simulink model "hevmodel"  (R2016b)
settings: Solver=VariableStepAuto  StartTime=0.0  StopTime=100.0  RelTol=1e-3
undefined symbols (not defined in the file): c_b_e1, c_b_E1, c_b_E2, c_b_e3, c_b_E3, c_b_E4, c_b_L1, c_b_L2, c_b_L3, c_b_L4, F, G, h, H_l, I_b_max, Mz, N, Q1, Q2, Q_b_0, rho_f, Ts, ubounds, w_eg_upper, w_em_upper, w_ice_upper
settings Model: Creator=Niklas  LastModifiedBy=Niklas
settings DataIOCC: SaveTime=off

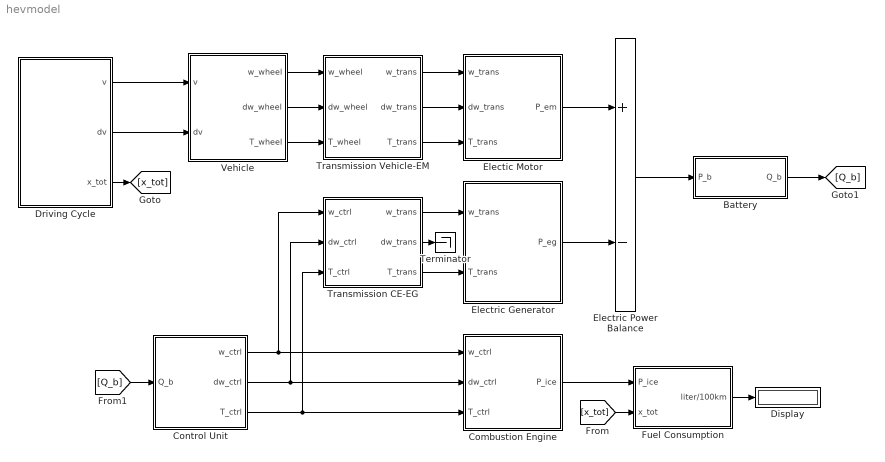
== system hevmodel ==
  Battery : Subsystem  mask{I_0=80, Q_b_IC_rel=50, t_ch=20}
      mask prompts: I_0 "Energy capacity of battery [Ah]"; Q_b_IC_rel "Initial charge of battery [%]"; t_ch "Current limit: minimum time to charge/discharge the battery [min]"
      mask init:
      | init_battery;
  Combustion Engine : Subsystem  mask{theta_ice=1, H_l=1, w_ice_idle=1, T_ice_idle=1, P_ice_idle=1, ENABLE_FUEL_CUTOFF=0, T_ice_cutoff=0, P_ice_cutoff=0}
      mask prompts: theta_ice "Engine inertia [kg*m^2]"; H_l "Fuel's lower heating value []"; w_ice_idle "Engine speed at idle [rad/s]"; T_ice_idle "Engine torque at idle [Nm]"; P_ice_idle "Engine power at idle [W]"; ENABLE_FUEL_CUTOFF "Enable fuel cutoff"; T_ice_cutoff "Engine torque at fuel cutoff [Nm]"; P_ice_cutoff "Engine power at fuel cutoff [W]"
  Control Unit : Subsystem
  Display : Display
  Driving Cycle : Subsystem  mask{Ts=0.1}
      mask prompts: Ts "Step size [s]"
      mask init:
      | init_drive_cycle
  Electic Motor : Subsystem  mask{theta_em=1}
      mask prompts: theta_em "Motor Ineratia [kg*m^2]"
      mask init:
      | init_EM
  Electric Generator : Subsystem
  Electric Power Balance : Sum  Inputs=+-
  Fuel Consumption : Subsystem
      mask init:
      | init_tank;
  Terminator : Terminator
  Transmission CE-EG : Subsystem  mask{gear_ratio=1, eta_gb=1, P_gb0=0, w_wheel_min=1}
      mask prompts: gear_ratio "Gear Ratio"; eta_gb "Efficiency"; P_gb0 "Idling losses (friction) [W]"; w_wheel_min "Minimum wheel speed beyond which losses are generated [rad/s]"
      mask init:
      | init_transmission;
  Transmission Vehicle-EM : Subsystem  mask{gear_ratio=0.707, eta_gb=0.975, P_gb0=0, w_wheel_min=1}
      mask prompts: gear_ratio "Gear Ratio"; eta_gb "Efficiency"; P_gb0 "Idling losses (friction) [W]"; w_wheel_min "Minimum wheel speed beyond which losses are generated [rad/s]"
      mask init:
      | init_transmission;
  Vehicle : Subsystem  mask{r_wheel=0.82, R0=554.9, R1=20.3, R2=3.56}
      mask prompts: r_wheel "Wheel Radius [m]"; R0 "Running Resistance R0 [N]"; R1 "Running Resistance R1 [N/(m/s)]"; R2 "Running Resistance R2 [N/(m/s)^2]"
      mask init:
      | init_vehicle
  wires:
  Transmission Vehicle-EM/1(w_trans) -> Electic Motor/1(w_trans)
  Transmission Vehicle-EM/2(dw_trans) -> Electic Motor/2(dw_trans)
  Transmission Vehicle-EM/3(T_trans) -> Electic Motor/3(T_trans)
  Vehicle/1(w_wheel) -> Transmission Vehicle-EM/1(w_wheel)
  Vehicle/2(dw_wheel) -> Transmission Vehicle-EM/2(dw_wheel)
  Vehicle/3(T_wheel) -> Transmission Vehicle-EM/3(T_wheel)
  Control Unit/1(w_ctrl) -> Transmission CE-EG/1(w_ctrl), Combustion Engine/1(w_ctrl)
  Control Unit/3(T_ctrl) -> Transmission CE-EG/3(T_ctrl), Combustion Engine/3(T_ctrl)
  Combustion Engine/1(P_ice) -> Fuel Consumption/1(P_ice)
  Fuel Consumption/1(liter/100km) -> Display/1
  Control Unit/2(dw_ctrl) -> Transmission CE-EG/2(dw_ctrl), Combustion Engine/2(dw_ctrl)
  Driving Cycle/1(v) -> Vehicle/1(v)
  Driving Cycle/2(dv) -> Vehicle/2(dv)
  Electric Power Balance/1 -> Battery/1(P_b)
  Electic Motor/1(P_em) -> Electric Power Balance/1
  Electric Generator/1(P_eg) -> Electric Power Balance/2
  Transmission CE-EG/1(w_trans) -> Electric Generator/1(w_trans)
  Transmission CE-EG/3(T_trans) -> Electric Generator/2(T_trans)
  Transmission CE-EG/2(dw_trans) -> Terminator/1
  Driving Cycle/3(x_tot) -> [x_tot]
  [x_tot] -> Fuel Consumption/2(x_tot)
  Battery/1(Q_b) -> [Q_b]
  [Q_b] -> Control Unit/1(Q_b)

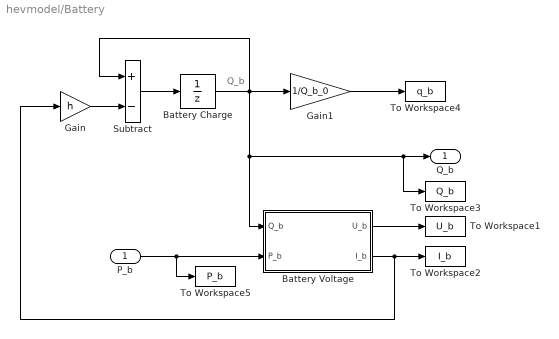
== system hevmodel/Battery ==
  note: Q_b
  P_b : Inport
  Battery Charge : UnitDelay  SampleTime=-1
  Battery Voltage : Subsystem
  Gain : Gain  Gain=h
  Gain1 : Gain  Gain=1/Q_b_0
  Subtract : Sum  Inputs=+-
  To Workspace1 : ToWorkspace  VariableName=U_b  SaveFormat=Timeseries  SampleTime=-1
  To Workspace2 : ToWorkspace  VariableName=I_b  SaveFormat=Timeseries  SampleTime=-1
  To Workspace3 : ToWorkspace  VariableName=Q_b  SaveFormat=Timeseries  SampleTime=-1
  To Workspace4 : ToWorkspace  VariableName=q_b  SaveFormat=Timeseries  SampleTime=-1
  To Workspace5 : ToWorkspace  VariableName=P_b  SaveFormat=Timeseries  SampleTime=-1
  Q_b : Outport
  wires:
  P_b/1 -> To Workspace5/1, Battery Voltage/2(P_b)
  Battery Charge/1 -> Subtract/1, Gain1/1, Battery Voltage/1(Q_b), To Workspace3/1, Q_b/1
  Subtract/1 -> Battery Charge/1
  Gain/1 -> Subtract/2
  Battery Voltage/2(I_b) -> To Workspace2/1, Gain/1
  Battery Voltage/1(U_b) -> To Workspace1/1
  Gain1/1 -> To Workspace4/1

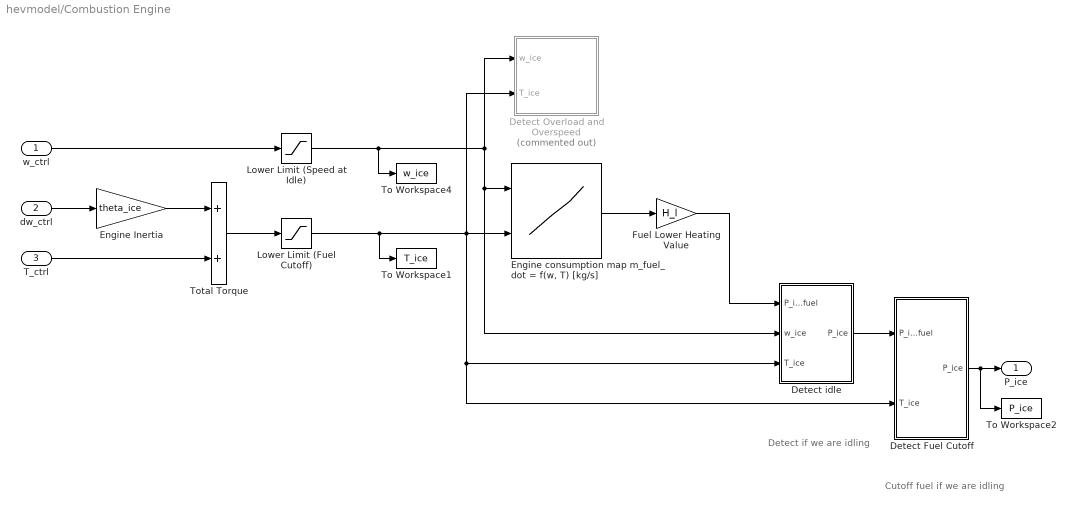
== system hevmodel/Combustion Engine ==
  note: Detect if we are idling
  note: Cutoff fuel if we are idling
  w_ctrl : Inport
  dw_ctrl : Inport  Port=2
  T_ctrl : Inport  Port=3
  Detect Fuel Cutoff : Subsystem
  Detect Overload and Overspeed : Subsystem  Commented=on
  Detect idle : Subsystem
  Engine Inertia : Gain  Gain=theta_ice
  "Engine consumption map m_fuel_dot = f(w, T) [kg/s]" : Lookup_n-D  BreakpointsForDimension1=[1:3]  BreakpointsForDimension2=[1:3]  InternalRulePriority=Speed  RndMeth=Simplest  InputSameDT=on
  Fuel Lower Heating Value : Gain  Gain=H_l
  Lower Limit (Fuel Cutoff) : Saturate  UpperLimit=inf  LowerLimit=T_ice_cutoff
  Lower Limit (Speed at Idle) : Saturate  UpperLimit=inf  LowerLimit=w_ice_idle
  To Workspace1 : ToWorkspace  VariableName=T_ice  SaveFormat=Timeseries  SampleTime=-1
  To Workspace2 : ToWorkspace  VariableName=P_ice  SaveFormat=Timeseries  SampleTime=-1
  To Workspace4 : ToWorkspace  VariableName=w_ice  SaveFormat=Timeseries  SampleTime=-1
  Total Torque : Sum
  P_ice : Outport
  wires:
  Detect Fuel Cutoff/1(P_ice) -> To Workspace2/1, P_ice/1
  dw_ctrl/1 -> Engine Inertia/1
  Engine Inertia/1 -> Total Torque/1
  T_ctrl/1 -> Total Torque/2
  Total Torque/1 -> Lower Limit (Fuel Cutoff)/1
  w_ctrl/1 -> Lower Limit (Speed at Idle)/1
  Lower Limit (Fuel Cutoff)/1 -> To Workspace1/1, Detect Overload and Overspeed/2(T_ice), Detect idle/3(T_ice), Detect Fuel Cutoff/2(T_ice), "Engine consumption map m_fuel_dot = f(w, T) [kg/s]"/2
  "Engine consumption map m_fuel_dot = f(w, T) [kg/s]"/1 -> Fuel Lower Heating Value/1
  Fuel Lower Heating Value/1 -> Detect idle/1(P_ice_fuel)
  Detect idle/1(P_ice) -> Detect Fuel Cutoff/1(P_ice_fuel)
  Lower Limit (Speed at Idle)/1 -> To Workspace4/1, Detect idle/2(w_ice), "Engine consumption map m_fuel_dot = f(w, T) [kg/s]"/1, Detect Overload and Overspeed/1(w_ice)

== system hevmodel/Control Unit ==
  Q_b : Inport
  Constant : Constant  Value=0
  MPC Controller : Subsystem  Commented=on  mask{F=F, G=G, M=Mz, N=N, Q1=Q1, Q2=Q2, ubounds=ubounds, Ts=Ts, ufname='solvempcproblem'}
      mask prompts: ubounds "Input bounds [u1min u1max;u2min u2max;...]"; ufname "Output function (Ex: 'myfun1')"
      mask Display:
      | port_label('input',1,'x')
      | port_label('output',1,'u')
  Terminator : Terminator
  w_ctrl : Outport
  dw_ctrl : Outport  Port=2
  T_ctrl : Outport  Port=3
  wires:
  Constant/1 -> T_ctrl/1, w_ctrl/1, dw_ctrl/1
  Q_b/1 -> Terminator/1

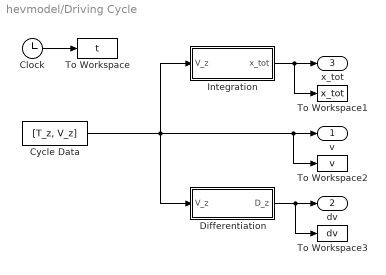
== system hevmodel/Driving Cycle ==
  Clock : Clock
  Cycle Data : FromWorkspace  VariableName=[T_z, V_z]  SampleTime=h
  Differentiation : Subsystem
  Integration : Subsystem
  To Workspace : ToWorkspace  VariableName=t  SampleTime=h
  To Workspace1 : ToWorkspace  VariableName=x_tot  SampleTime=-1
  To Workspace2 : ToWorkspace  VariableName=v  SampleTime=-1
  To Workspace3 : ToWorkspace  VariableName=dv  SampleTime=-1
  v : Outport
  dv : Outport  Port=2
  x_tot : Outport  Port=3
  wires:
  Clock/1 -> To Workspace/1
  Cycle Data/1 -> Differentiation/1(V_z), Integration/1(V_z), To Workspace2/1, v/1
  Integration/1(x_tot) -> To Workspace1/1, x_tot/1
  Differentiation/1(D_z) -> To Workspace3/1, dv/1

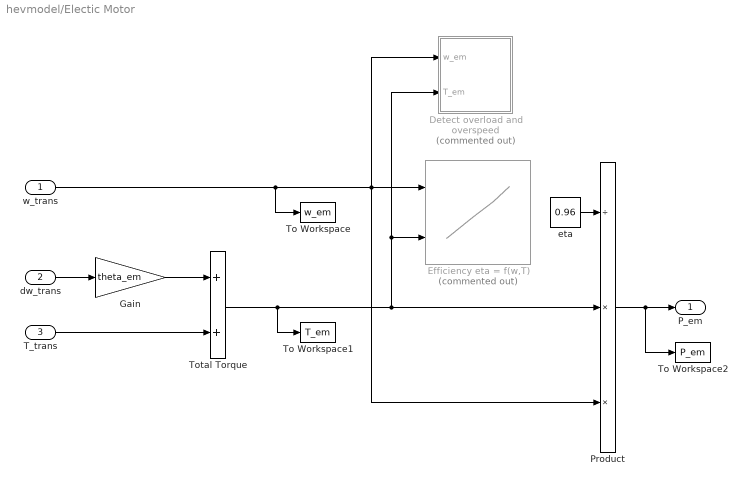
== system hevmodel/Electic Motor ==
  w_trans : Inport
  dw_trans : Inport  Port=2
  T_trans : Inport  Port=3
  Detect overload and overspeed : Subsystem  Commented=on
  Efficiency eta = f(w,T) : Lookup_n-D  Commented=on  BreakpointsForDimension1=[1:3]  BreakpointsForDimension2=[1:3]  InternalRulePriority=Speed  RndMeth=Simplest  InputSameDT=on
  Gain : Gain  Gain=theta_em
  Product : Product  Inputs=/**
  To Workspace : ToWorkspace  VariableName=w_em  SaveFormat=Timeseries  SampleTime=-1
  To Workspace1 : ToWorkspace  VariableName=T_em  SaveFormat=Timeseries  SampleTime=-1
  To Workspace2 : ToWorkspace  VariableName=P_em  SaveFormat=Timeseries  SampleTime=-1
  Total Torque : Sum
  eta : Constant  Value=0.96
  P_em : Outport
  wires:
  Product/1 -> To Workspace2/1, P_em/1
  dw_trans/1 -> Gain/1
  Gain/1 -> Total Torque/1
  T_trans/1 -> Total Torque/2
  Total Torque/1 -> To Workspace1/1, Efficiency eta = f(w,T)/2, Detect overload and overspeed/2(T_em), Product/2
  w_trans/1 -> To Workspace/1, Product/3, Detect overload and overspeed/1(w_em), Efficiency eta = f(w,T)/1
  eta/1 -> Product/1

== system hevmodel/Electric Generator ==
  w_trans : Inport
  T_trans : Inport  Port=2
  Detect overload and overspeed : Subsystem  Commented=on
  Efficiency eta = f(w,T) : Lookup_n-D  Commented=on  BreakpointsForDimension1=[1:3]  BreakpointsForDimension2=[1:3]  InternalRulePriority=Speed  RndMeth=Simplest  InputSameDT=on
  Product : Product  Inputs=3
  To Workspace1 : ToWorkspace  VariableName=w_eg  SaveFormat=Timeseries  SampleTime=-1
  To Workspace2 : ToWorkspace  VariableName=T_eg  SaveFormat=Timeseries  SampleTime=-1
  To Workspace3 : ToWorkspace  VariableName=P_eg  SaveFormat=Timeseries  SampleTime=-1
  eta : Constant  Value=0.96
  P_eg : Outport
  wires:
  Product/1 -> To Workspace3/1, P_eg/1
  T_trans/1 -> To Workspace2/1, Efficiency eta = f(w,T)/2, Detect overload and overspeed/2(T_eg), Product/2
  w_trans/1 -> To Workspace1/1, Product/3, Detect overload and overspeed/1(w_eg), Efficiency eta = f(w,T)/1
  eta/1 -> Product/1

== system hevmodel/Fuel Consumption ==
  P_ice : Inport
  x_tot : Inport  Port=2
  Divide : Product  Inputs=*/
  Gain : Gain  Gain=1/rho_f
  Gain1 : Gain  Gain=1e5
  Integration : Subsystem
  Saturation : Saturate  UpperLimit=inf  LowerLimit=1
  liter/100km : Outport
  wires:
  P_ice/1 -> Integration/1(P_ice)
  Gain1/1 -> liter/100km/1
  Integration/1(m_fuel) -> Gain/1
  Gain/1 -> Divide/1
  Divide/1 -> Gain1/1
  x_tot/1 -> Saturation/1
  Saturation/1 -> Divide/2

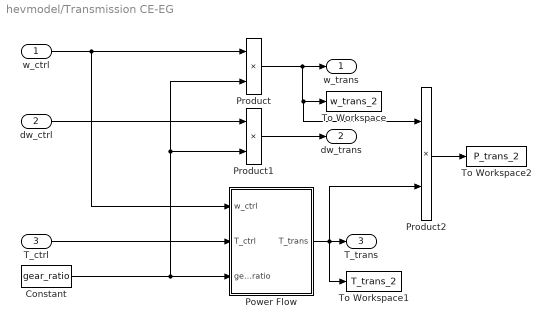
== system hevmodel/Transmission CE-EG ==
  w_ctrl : Inport
  dw_ctrl : Inport  Port=2
  T_ctrl : Inport  Port=3
  Constant : Constant  Value=gear_ratio
  Power Flow : Subsystem
  Product : Product
  Product1 : Product
  Product2 : Product
  To Workspace : ToWorkspace  VariableName=w_trans_2  SaveFormat=Timeseries  SampleTime=-1
  To Workspace1 : ToWorkspace  VariableName=T_trans_2  SaveFormat=Timeseries  SampleTime=-1
  To Workspace2 : ToWorkspace  VariableName=P_trans_2  SaveFormat=Timeseries  SampleTime=-1
  w_trans : Outport
  dw_trans : Outport  Port=2
  T_trans : Outport  Port=3
  wires:
  w_ctrl/1 -> Product/1, Power Flow/1(w_ctrl)
  dw_ctrl/1 -> Product1/1
  Product/1 -> Product2/1, To Workspace/1, w_trans/1
  Power Flow/1(T_trans) -> To Workspace1/1, Product2/2, T_trans/1
  Product1/1 -> dw_trans/1
  T_ctrl/1 -> Power Flow/2(T_ctrl)
  Constant/1 -> Product/2, Product1/2, Power Flow/3(gear_ratio)
  Product2/1 -> To Workspace2/1

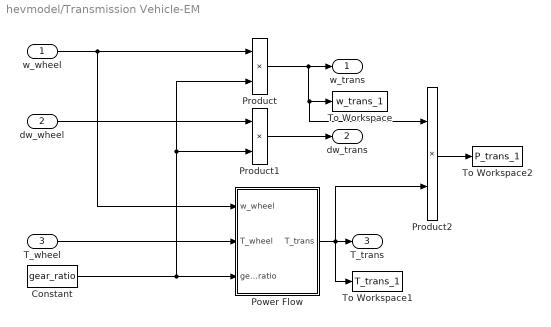
== system hevmodel/Transmission Vehicle-EM ==
  w_wheel : Inport
  dw_wheel : Inport  Port=2
  T_wheel : Inport  Port=3
  Constant : Constant  Value=gear_ratio
  Power Flow : Subsystem
  Product : Product
  Product1 : Product
  Product2 : Product
  To Workspace : ToWorkspace  VariableName=w_trans_1  SaveFormat=Timeseries  SampleTime=-1
  To Workspace1 : ToWorkspace  VariableName=T_trans_1  SaveFormat=Timeseries  SampleTime=-1
  To Workspace2 : ToWorkspace  VariableName=P_trans_1  SaveFormat=Timeseries  SampleTime=-1
  w_trans : Outport
  dw_trans : Outport  Port=2
  T_trans : Outport  Port=3
  wires:
  w_wheel/1 -> Product/1, Power Flow/1(w_wheel)
  dw_wheel/1 -> Product1/1
  Product/1 -> Product2/1, To Workspace/1, w_trans/1
  Power Flow/1(T_trans) -> To Workspace1/1, Product2/2, T_trans/1
  Product1/1 -> dw_trans/1
  T_wheel/1 -> Power Flow/2(T_wheel)
  Constant/1 -> Product/2, Product1/2, Power Flow/3(gear_ratio)
  Product2/1 -> To Workspace2/1

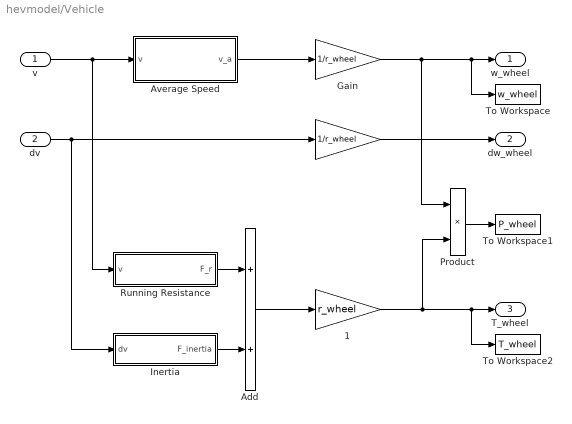
== system hevmodel/Vehicle ==
  v : Inport
  dv : Inport  Port=2
  " " : Gain  Gain=1/r_wheel
  " 1" : Gain  Gain=r_wheel
  Add : Sum
  Average Speed : Subsystem
  Gain : Gain  Gain=1/r_wheel
  Inertia : Subsystem
  Product : Product
  Running Resistance : Subsystem
  To Workspace : ToWorkspace  VariableName=w_wheel  SaveFormat=Timeseries  SampleTime=-1
  To Workspace1 : ToWorkspace  VariableName=P_wheel  SaveFormat=Timeseries  SampleTime=-1
  To Workspace2 : ToWorkspace  VariableName=T_wheel  SaveFormat=Timeseries  SampleTime=-1
  w_wheel : Outport
  dw_wheel : Outport  Port=2
  T_wheel : Outport  Port=3
  wires:
  v/1 -> Running Resistance/1(v), Average Speed/1(v)
  Gain/1 -> To Workspace/1, w_wheel/1, Product/1
  " "/1 -> dw_wheel/1
  dv/1 -> Inertia/1(dv), " "/1
  " 1"/1 -> To Workspace2/1, T_wheel/1, Product/2
  Product/1 -> To Workspace1/1
  Average Speed/1(v_a) -> Gain/1
  Add/1 -> " 1"/1
  Inertia/1(F_inertia) -> Add/2
  Running Resistance/1(F_r) -> Add/1

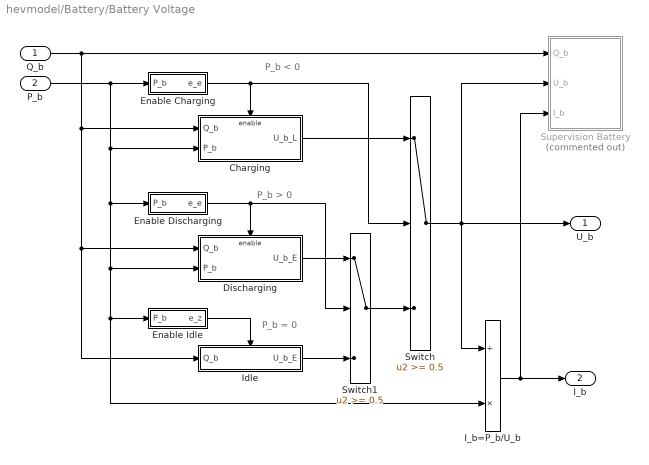
== system hevmodel/Battery/Battery Voltage ==
  note: P_b < 0
  note: P_b = 0
  note: P_b > 0
  Q_b : Inport
  P_b : Inport  Port=2
  Charging : Subsystem
  Discharging : Subsystem
  Enable Charging : Subsystem
  Enable Discharging : Subsystem
  Enable Idle : Subsystem
  I_b=P_b/U_b : Product  Inputs=/*
  Idle : Subsystem
  Supervision Battery : Subsystem  Commented=on
  Switch : Switch  Threshold=0.5
  Switch1 : Switch  Threshold=0.5
  U_b : Outport
  I_b : Outport  Port=2
  wires:
  Q_b/1 -> Charging/1(Q_b), Idle/1(Q_b), Discharging/1(Q_b), Supervision Battery/1(Q_b)
  Enable Charging/1(e_e) -> Switch/2, Charging/Enable
  I_b=P_b/U_b/1 -> I_b/1, Supervision Battery/3(I_b)
  P_b/1 -> I_b=P_b/U_b/2, Enable Idle/1(P_b), Discharging/2(P_b), Enable Discharging/1(P_b), Charging/2(P_b), Enable Charging/1(P_b)
  Enable Idle/1(e_z) -> Idle/Enable
  Enable Discharging/1(e_e) -> Switch1/2, Discharging/Enable
  Discharging/1(U_b_E) -> Switch1/1
  Switch1/1 -> Switch/3
  Idle/1(U_b_E) -> Switch1/3
  Switch/1 -> I_b=P_b/U_b/1, Supervision Battery/2(U_b), U_b/1
  Charging/1(U_b_L) -> Switch/1

== system hevmodel/Combustion Engine/Detect Fuel Cutoff ==
  P_ice_fuel : Inport
  T_ice : Inport  Port=2
  Constant : Constant  Value=P_ice_cutoff
  Constant1 : Constant  Value=ENABLE_FUEL_CUTOFF
  Switch1 : Switch  Threshold=T_ice_cutoff + 0.01
  Switch2 : Switch  Threshold=0.5
  P_ice : Outport
  wires:
  Switch2/1 -> P_ice/1
  T_ice/1 -> Switch1/2
  P_ice_fuel/1 -> Switch2/3, Switch1/1
  Constant/1 -> Switch1/3
  Constant1/1 -> Switch2/2
  Switch1/1 -> Switch2/1

== system hevmodel/Combustion Engine/Detect Overload and Overspeed ==
  w_ice : Inport
  T_ice : Inport  Port=2
  Abs : Abs
  Constant : Constant  Value=w_ice_upper
  Maximum Torque : Lookup_n-D  NumberOfTableDimensions=1  BreakpointsForDimension1=[-5:5]  Table=tanh([-5:5])  InternalRulePriority=Speed  RndMeth=Simplest  InputSameDT=on
  Saturation : Saturate  UpperLimit=0  LowerLimit=-inf
  Saturation1 : Saturate  UpperLimit=0  LowerLimit=-inf
  Stop Simulation : Stop
  Stop Simulation1 : Stop
  Subtract1 : Sum  Inputs=+-
  Subtract2 : Sum  Inputs=+-
  wires:
  Maximum Torque/1 -> Subtract1/1
  Subtract1/1 -> Saturation/1
  Saturation/1 -> Stop Simulation/1
  Abs/1 -> Subtract1/2
  w_ice/1 -> Subtract2/2, Maximum Torque/1
  T_ice/1 -> Abs/1
  Constant/1 -> Subtract2/1
  Saturation1/1 -> Stop Simulation1/1
  Subtract2/1 -> Saturation1/1

== system hevmodel/Combustion Engine/Detect idle ==
  P_ice_fuel : Inport
  w_ice : Inport  Port=2
  T_ice : Inport  Port=3
  Constant : Constant  Value=P_ice_idle
  Idle detection : Fcn  Expr=(u(1) <= w_ice_idle) * (u(2) <= T_ice_idle)
  Mux : Mux  Inputs=2
  Switch : Switch  Criteria=u2 > Threshold
  P_ice : Outport
  wires:
  w_ice/1 -> Mux/1
  T_ice/1 -> Mux/2
  Switch/1 -> P_ice/1
  P_ice_fuel/1 -> Switch/3
  Constant/1 -> Switch/1
  Idle detection/1 -> Switch/2
  Mux/1 -> Idle detection/1

== system hevmodel/Control Unit/MPC Controller ==
  In1 : Inport
  Clock : Clock
  MPC Controller1 : M-S-Function  FunctionName=mympccontroller  Parameters=F,G,M,N,Q1,Q2,ubounds,Ts,ufname  mask{F=F, G=G, M=M, N=N, Q1=Q1, Q2=Q2, ubounds=ubounds, Ts=Ts, ufname=ufname}
      mask prompts: ubounds "ubounds [u1min u1max;u2min u2max;...]"; ufname "Output function (Ex: 'myfun1')"
      mask Display:
      | port_label('input',1,'x')
      | port_label('input',2,'t')
      | port_label('output',1,'u')
  Out1 : Outport
  wires:
  Clock/1 -> MPC Controller1/2
  In1/1 -> MPC Controller1/1
  MPC Controller1/1 -> Out1/1

== system hevmodel/Driving Cycle/Differentiation ==
  V_z : Inport
  Add : Sum  Inputs=+-
  Unit Delay : UnitDelay  SampleTime=-1
  D_z : Outport
  wires:
  Unit Delay/1 -> Add/2
  V_z/1 -> Unit Delay/1, Add/1
  Add/1 -> D_z/1

== system hevmodel/Driving Cycle/Integration ==
  V_z : Inport
  Add : Sum
  Add1 : Sum
  Gain : Gain  Gain=0.5*h
  Unit Delay : UnitDelay  SampleTime=-1
  Unit Delay1 : UnitDelay  SampleTime=-1
  x_tot : Outport
  wires:
  Unit Delay/1 -> Add/2
  V_z/1 -> Add/1, Unit Delay/1
  Add/1 -> Gain/1
  Gain/1 -> Add1/2
  Add1/1 -> Unit Delay1/1
  Unit Delay1/1 -> x_tot/1, Add1/1

== system hevmodel/Electic Motor/Detect overload and overspeed ==
  w_em : Inport
  T_em : Inport  Port=2
  Abs : Abs
  Add : Sum  Inputs=+-
  Add1 : Sum  Inputs=+-
  Constant : Constant  Value=w_em_upper
  Maximum Torque : Lookup_n-D  NumberOfTableDimensions=1  BreakpointsForDimension1=[-5:5]  Table=tanh([-5:5])  InternalRulePriority=Speed  RndMeth=Simplest  InputSameDT=on
  Saturation : Saturate  UpperLimit=0  LowerLimit=-inf
  Saturation1 : Saturate  UpperLimit=0  LowerLimit=-inf
  Stop Simulation : Stop
  Stop Simulation1 : Stop
  wires:
  w_em/1 -> Add1/2, Maximum Torque/1
  T_em/1 -> Abs/1
  Maximum Torque/1 -> Add/1
  Abs/1 -> Add/2
  Add/1 -> Saturation/1
  Saturation/1 -> Stop Simulation1/1
  Constant/1 -> Add1/1
  Add1/1 -> Saturation1/1
  Saturation1/1 -> Stop Simulation/1

== system hevmodel/Electric Generator/Detect overload and overspeed ==
  w_eg : Inport
  T_eg : Inport  Port=2
  Abs : Abs
  Add : Sum  Inputs=+-
  Add1 : Sum  Inputs=+-
  Constant : Constant  Value=w_eg_upper
  Maximum Torque : Lookup_n-D  NumberOfTableDimensions=1  BreakpointsForDimension1=[-5:5]  Table=tanh([-5:5])  InternalRulePriority=Speed  RndMeth=Simplest  InputSameDT=on
  Saturation : Saturate  UpperLimit=0  LowerLimit=-inf
  Saturation1 : Saturate  UpperLimit=0  LowerLimit=-inf
  Stop Simulation : Stop
  Stop Simulation1 : Stop
  wires:
  w_eg/1 -> Add1/2, Maximum Torque/1
  T_eg/1 -> Abs/1
  Maximum Torque/1 -> Add/1
  Abs/1 -> Add/2
  Add/1 -> Saturation/1
  Saturation/1 -> Stop Simulation1/1
  Constant/1 -> Add1/1
  Add1/1 -> Saturation1/1
  Saturation1/1 -> Stop Simulation/1

== system hevmodel/Fuel Consumption/Integration ==
  P_ice : Inport
  Add1 : Sum
  Add2 : Sum
  Constant : Constant  Value=1/H_l
  Fuel Consumption : UnitDelay  SampleTime=-1
  Gain : Gain  Gain=0.5*h
  Product : Product
  To Workspace1 : ToWorkspace  VariableName=m_dot_fuel  SaveFormat=Timeseries  SampleTime=-1
  To Workspace2 : ToWorkspace  VariableName=m_fuel  SaveFormat=Timeseries  SampleTime=-1
  Unit Delay : UnitDelay  SampleTime=-1
  m_fuel : Outport
  wires:
  Fuel Consumption/1 -> To Workspace2/1, m_fuel/1, Add1/1
  Add1/1 -> Fuel Consumption/1
  P_ice/1 -> Add2/1, Unit Delay/1
  Unit Delay/1 -> Add2/2
  Constant/1 -> Product/1
  Add2/1 -> Gain/1
  Gain/1 -> Product/2
  Product/1 -> To Workspace1/1, Add1/2

== system hevmodel/Transmission CE-EG/Power Flow ==
  w_ctrl : Inport
  T_ctrl : Inport  Port=2
  gear_ratio : Inport  Port=3
  Subsystem : Subsystem
  Subsystem1 : Subsystem
  Switch : Switch
  T_trans : Outport
  wires:
  T_ctrl/1 -> Subsystem1/2(T_ctrl), Subsystem/2(T_ctrl), Switch/2
  Switch/1 -> T_trans/1
  Subsystem1/1(T_trans-) -> Switch/3
  Subsystem/1(T_trans+) -> Switch/1
  gear_ratio/1 -> Subsystem1/3(gear_ratio), Subsystem/3(gear_ratio)
  w_ctrl/1 -> Subsystem1/1(w_ctrl), Subsystem/1(w_ctrl)

== system hevmodel/Transmission Vehicle-EM/Power Flow ==
  w_wheel : Inport
  T_wheel : Inport  Port=2
  gear_ratio : Inport  Port=3
  "Energy Engine -> Wheel" : Subsystem
  "Energy Wheel -> Engine" : Subsystem
  Switch : Switch
  T_trans : Outport
  wires:
  T_wheel/1 -> "Energy Wheel -> Engine"/2(T_wheel), "Energy Engine -> Wheel"/2(T_wheel), Switch/2
  Switch/1 -> T_trans/1
  "Energy Wheel -> Engine"/1(T_trans-) -> Switch/3
  "Energy Engine -> Wheel"/1(T_trans+) -> Switch/1
  gear_ratio/1 -> "Energy Wheel -> Engine"/3(gear_ratio), "Energy Engine -> Wheel"/3(gear_ratio)
  w_wheel/1 -> "Energy Wheel -> Engine"/1(w_wheel), "Energy Engine -> Wheel"/1(w_wheel)

== system hevmodel/Vehicle/Average Speed ==
  v : Inport
  Add : Sum
  Gain : Gain  Gain=0.5
  Unit Delay : UnitDelay  SampleTime=-1
  v_a : Outport
  wires:
  v/1 -> Unit Delay/1, Add/1
  Unit Delay/1 -> Add/2
  Add/1 -> Gain/1
  Gain/1 -> v_a/1

== system hevmodel/Vehicle/Inertia ==
  dv : Inport
  Inertia : Fcn  Expr=39600*(1.08)*u/h
  F_inertia : Outport
  wires:
  dv/1 -> Inertia/1
  Inertia/1 -> F_inertia/1

== system hevmodel/Vehicle/Running Resistance ==
  v : Inport
  Running Resistance : Fcn  Expr=R2*u^2+R1*u+R0
  Standstill : Constant  Value=0
  Switch : Switch  Criteria=u2 > Threshold
  F_r : Outport
  wires:
  Running Resistance/1 -> Switch/1
  v/1 -> Switch/2, Running Resistance/1
  Switch/1 -> F_r/1
  Standstill/1 -> Switch/3

== system hevmodel/Battery/Battery Voltage/Charging ==
  note: P_b/I_0
  note: 1- q
  Q_b : Inport
  P_b : Inport  Port=2
  Enable : EnablePort
  Constant : Constant  Value=Q_b_0
  Fcn1 : Fcn  Expr=(c_b_L3*u[1]+c_b_L1+sqrt((c_b_L3*u[1]+c_b_L1)^2+4*(c_b_L4*u[1]+c_b_L2)*(-u[2])))/2
  Gain : Gain  Gain=1/Q_b_0
  Gain1 : Gain  Gain=1/I_0
  Mux : Mux  Inputs=2
  Subtract : Sum  Inputs=-+
  U_b_L : Outport
  wires:
  P_b/1 -> Gain1/1
  Gain1/1 -> Mux/2
  Gain/1 -> Mux/1
  Subtract/1 -> Gain/1
  Constant/1 -> Subtract/2
  Q_b/1 -> Subtract/1
  Fcn1/1 -> U_b_L/1
  Mux/1 -> Fcn1/1

== system hevmodel/Battery/Battery Voltage/Discharging ==
  note: P/I_0
  note: 1-q
  Q_b : Inport
  P_b : Inport  Port=2
  Enable : EnablePort
  Constant : Constant  Value=Q_b_0
  Fcn : Fcn  Expr=(c_b_E3*u[1]+c_b_E1+sqrt((c_b_E3*u[1]+c_b_E1)^2+4*(c_b_E4*u[1]+c_b_E2)*(-u[2])))/2
  Gain : Gain  Gain=1/Q_b_0
  Gain1 : Gain  Gain=1/I_0
  Mux : Mux  Inputs=2
  Subtract : Sum  Inputs=-+
  U_b_E : Outport
  wires:
  Gain1/1 -> Mux/2
  Gain/1 -> Mux/1
  Subtract/1 -> Gain/1
  Constant/1 -> Subtract/2
  Fcn/1 -> U_b_E/1
  Mux/1 -> Fcn/1
  Q_b/1 -> Subtract/1
  P_b/1 -> Gain1/1

== system hevmodel/Battery/Battery Voltage/Enable Charging ==
  P_b : Inport
  Gain : Gain  Gain=-1
  Saturation : Saturate  UpperLimit=0  LowerLimit=-inf
  Sign : Signum
  e_e : Outport
  wires:
  Sign/1 -> e_e/1
  P_b/1 -> Saturation/1
  Saturation/1 -> Gain/1
  Gain/1 -> Sign/1

== system hevmodel/Battery/Battery Voltage/Enable Discharging ==
  P_b : Inport
  Saturation : Saturate  UpperLimit=inf  LowerLimit=0
  Sign : Signum
  e_e : Outport
  wires:
  Sign/1 -> e_e/1
  Saturation/1 -> Sign/1
  P_b/1 -> Saturation/1

== system hevmodel/Battery/Battery Voltage/Enable Idle ==
  P_b : Inport
  Abs : Abs
  Constant : Constant
  Sign : Signum
  Subtract : Sum  Inputs=-+
  e_z : Outport
  wires:
  Subtract/1 -> e_z/1
  Sign/1 -> Abs/1
  P_b/1 -> Sign/1
  Constant/1 -> Subtract/2
  Abs/1 -> Subtract/1

== system hevmodel/Battery/Battery Voltage/Idle ==
  note: (1 - q) * c_b_L3 + c_b_L1
  Q_b : Inport
  Enable : EnablePort
  Add : Sum
  Add1 : Sum  Inputs=-+
  Constant : Constant  Value=Q_b_0
  Constant1 : Constant  Value=c_b_L1
  Gain4 : Gain  Gain=c_b_L3/Q_b_0  SaturateOnIntegerOverflow=on  OutDataTypeStr=Inherit: Same as input  ParamDataTypeStr=Inherit: Same as input
  U_b_E : Outport
  wires:
  Q_b/1 -> Add1/1
  Constant1/1 -> Add/2
  Constant/1 -> Add1/2
  Add/1 -> U_b_E/1
  Add1/1 -> Gain4/1
  Gain4/1 -> Add/1

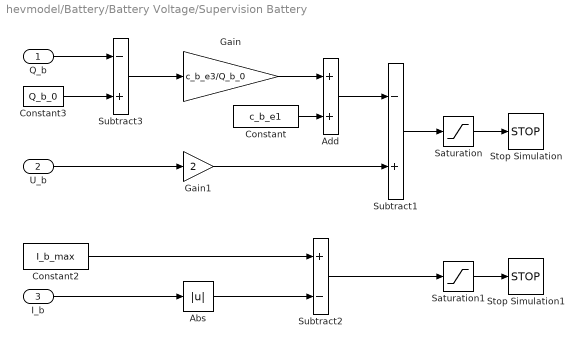
== system hevmodel/Battery/Battery Voltage/Supervision Battery ==
  Q_b : Inport
  U_b : Inport  Port=2
  I_b : Inport  Port=3
  Abs : Abs
  Add : Sum
  Constant : Constant  Value=c_b_e1
  Constant2 : Constant  Value=I_b_max
  Constant3 : Constant  Value=Q_b_0
  Gain : Gain  Gain=c_b_e3/Q_b_0
  Gain1 : Gain  Gain=2
  Saturation : Saturate
  Saturation1 : Saturate
  Stop Simulation : Stop
  Stop Simulation1 : Stop
  Subtract1 : Sum  Inputs=-+
  Subtract2 : Sum  Inputs=+-
  Subtract3 : Sum  Inputs=-+
  wires:
  Q_b/1 -> Subtract3/1
  Constant3/1 -> Subtract3/2
  Subtract3/1 -> Gain/1
  Gain/1 -> Add/1
  Constant/1 -> Add/2
  Add/1 -> Subtract1/1
  Subtract1/1 -> Saturation/1
  Saturation/1 -> Stop Simulation/1
  Gain1/1 -> Subtract1/2
  U_b/1 -> Gain1/1
  I_b/1 -> Abs/1
  Abs/1 -> Subtract2/2
  Constant2/1 -> Subtract2/1
  Saturation1/1 -> Stop Simulation1/1
  Subtract2/1 -> Saturation1/1

== system hevmodel/Transmission CE-EG/Power Flow/Subsystem ==
  w_ctrl : Inport
  T_ctrl : Inport  Port=2
  gear_ratio : Inport  Port=3
  Add : Sum
  Constant : Constant  Value=inf
  Constant1 : Constant  Value=P_gb0
  Divide : Product  Inputs=*/
  Divide1 : Product  Inputs=/*
  Gain : Gain  Gain=eta_gb
  Switch : Switch  Threshold=w_wheel_min
  T_trans+ : Outport
  wires:
  Divide/1 -> T_trans+/1
  Add/1 -> Divide/1
  Divide1/1 -> Add/1
  Switch/1 -> Divide1/1
  w_ctrl/1 -> Switch/1, Switch/2
  Constant/1 -> Switch/3
  T_ctrl/1 -> Add/2
  Constant1/1 -> Divide1/2
  Gain/1 -> Divide/2
  gear_ratio/1 -> Gain/1

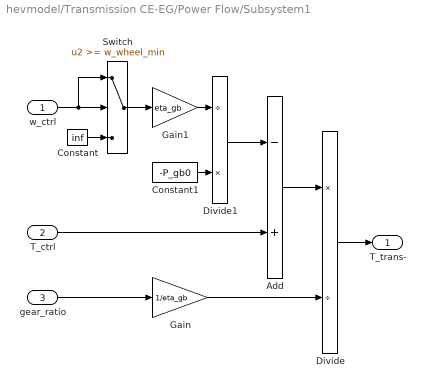
== system hevmodel/Transmission CE-EG/Power Flow/Subsystem1 ==
  w_ctrl : Inport
  T_ctrl : Inport  Port=2
  gear_ratio : Inport  Port=3
  Add : Sum  Inputs=-+
  Constant : Constant  Value=inf
  Constant1 : Constant  Value=-P_gb0
  Divide : Product  Inputs=*/
  Divide1 : Product  Inputs=/*
  Gain : Gain  Gain=1/eta_gb
  Gain1 : Gain  Gain=eta_gb
  Switch : Switch  Threshold=w_wheel_min
  T_trans- : Outport
  wires:
  Divide/1 -> T_trans-/1
  Add/1 -> Divide/1
  Divide1/1 -> Add/1
  w_ctrl/1 -> Switch/1, Switch/2
  Constant/1 -> Switch/3
  T_ctrl/1 -> Add/2
  Constant1/1 -> Divide1/2
  Gain/1 -> Divide/2
  gear_ratio/1 -> Gain/1
  Switch/1 -> Gain1/1
  Gain1/1 -> Divide1/1

== system hevmodel/Transmission Vehicle-EM/Power Flow/Energy Engine -> Wheel ==
  w_wheel : Inport
  T_wheel : Inport  Port=2
  gear_ratio : Inport  Port=3
  Add : Sum
  Constant : Constant  Value=inf
  Constant1 : Constant  Value=P_gb0
  Divide : Product  Inputs=*/
  Divide1 : Product  Inputs=/*
  Gain : Gain  Gain=eta_gb
  Switch : Switch  Threshold=w_wheel_min
  T_trans+ : Outport
  wires:
  Divide/1 -> T_trans+/1
  Add/1 -> Divide/1
  Divide1/1 -> Add/1
  Switch/1 -> Divide1/1
  w_wheel/1 -> Switch/1, Switch/2
  Constant/1 -> Switch/3
  T_wheel/1 -> Add/2
  Constant1/1 -> Divide1/2
  Gain/1 -> Divide/2
  gear_ratio/1 -> Gain/1

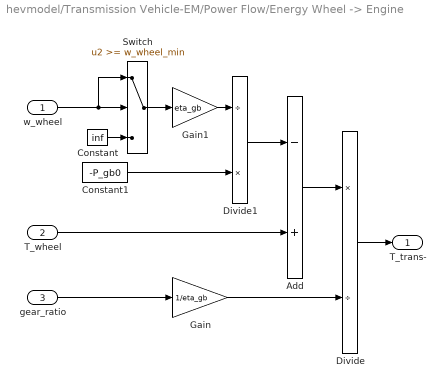
== system hevmodel/Transmission Vehicle-EM/Power Flow/Energy Wheel -> Engine ==
  w_wheel : Inport
  T_wheel : Inport  Port=2
  gear_ratio : Inport  Port=3
  Add : Sum  Inputs=-+
  Constant : Constant  Value=inf
  Constant1 : Constant  Value=-P_gb0
  Divide : Product  Inputs=*/
  Divide1 : Product  Inputs=/*
  Gain : Gain  Gain=1/eta_gb
  Gain1 : Gain  Gain=eta_gb
  Switch : Switch  Threshold=w_wheel_min
  T_trans- : Outport
  wires:
  Divide/1 -> T_trans-/1
  Add/1 -> Divide/1
  Divide1/1 -> Add/1
  w_wheel/1 -> Switch/1, Switch/2
  Constant/1 -> Switch/3
  T_wheel/1 -> Add/2
  Constant1/1 -> Divide1/2
  Gain/1 -> Divide/2
  gear_ratio/1 -> Gain/1
  Switch/1 -> Gain1/1
  Gain1/1 -> Divide1/1
